simulink model "SOC_Estimation"  (R2024b)
settings: configuration reference "BMS_Sw_CodeGenConfig" (kept outside this file)
undefined symbols (not defined in the file): BatteryNN, BMS_State_Enum, DiscIntNeverNeededParam, Np_Module, Ns_Module, NumModules, SOCInit
libraries: simulink x1, BatteryEstimators x1
settings Model: DataDictionary=DD_SOC_Estimation.sldd  ExtModeTrigDuration=5  Creator=cpatel  LastModifiedBy=97433
settings ConfigSetRef: SourceName=BMS_Sw_CodeGenConfig

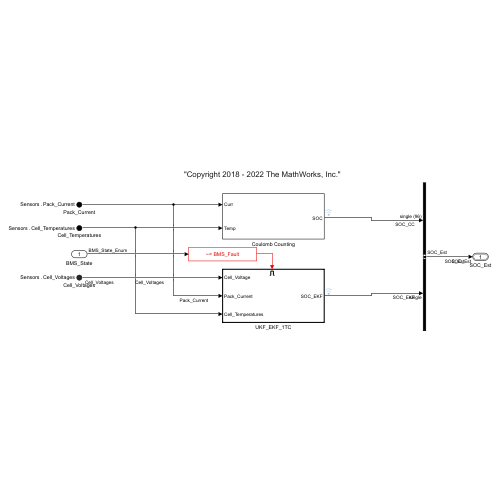
[thumbnail: Simulink's stored preview of the top-level diagram]
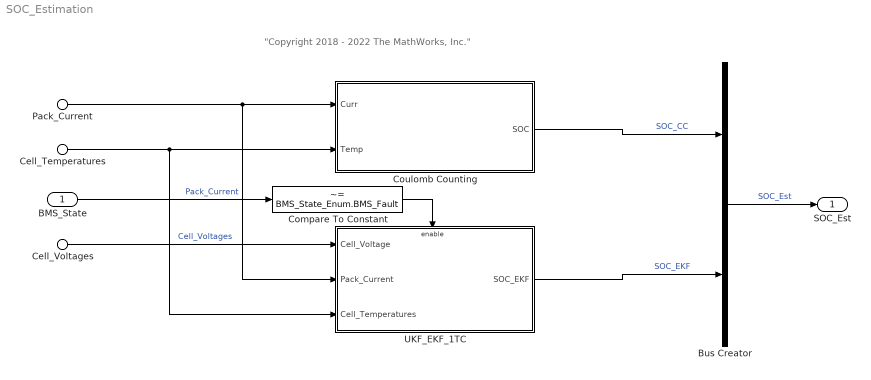
== system SOC_Estimation ==
  note: "Copyright 2018 - 2022 The MathWorks, Inc."
  BMS_State : Inport  OutDataTypeStr=Enum: BMS_State_Enum
  Cell_Voltages : Inport  Port=2  PortName=Sensors  Element=Cell_Voltages
  Pack_Current : Inport  Port=2  PortName=Sensors  Element=Pack_Current
  Cell_Temperatures : Inport  Port=2  PortName=Sensors  Element=Cell_Temperatures
  Bus Creator : BusCreator  Inputs=2  OutDataTypeStr=Bus: SOC_Est  NonVirtualBus=on
      settings: InheritFromInputs=off
  Compare To Constant : simulink/Logic and Bit Operations/Compare To Constant  relop=~=  const=BMS_State_Enum.BMS_Fault  OutDataTypeStr=boolean
  Coulomb Counting : Subsystem  VariantControl=SocAlgo==1
  UKF_EKF_1TC : Subsystem  VariantControl=CellType==1
  SOC_Est : Outport  OutDataTypeStr=Bus: SOC_Est  SampleTime=[0.10000000000000001,0]  VectorParamsAs1DForOutWhenUnconnected=off  BusOutputAsStruct=on
  wires:
  Cell_Voltages/1 -> UKF_EKF_1TC/1(Cell_Voltage)  "Cell_Voltages"
  Bus Creator/1 -> SOC_Est/1  "SOC_Est"
  Coulomb Counting/1(SOC) -> Bus Creator/1  "SOC_CC"
  UKF_EKF_1TC/1(SOC_EKF) -> Bus Creator/2  "SOC_EKF"
  BMS_State/1 -> Compare To Constant/1
  Compare To Constant/1 -> UKF_EKF_1TC/Enable
  Pack_Current/1 -> UKF_EKF_1TC/2(Pack_Current), Coulomb Counting/1(Curr)  "Pack_Current"
  Cell_Temperatures/1 -> Coulomb Counting/2(Temp), UKF_EKF_1TC/3(Cell_Temperatures)

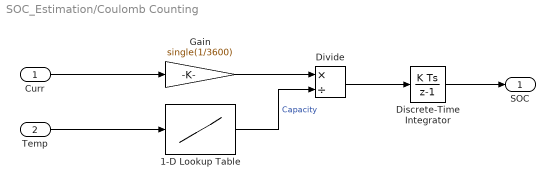
== system SOC_Estimation/Coulomb Counting ==
  Curr : Inport
  Temp : Inport  Port=2
  1-D Lookup Table : Lookup_n-D  NumberOfTableDimensions=1  BreakpointsForDimension1=single(BatteryNN(1).T_vec)  Table=single(BatteryNN(1).AH)*Np_Module  InternalRulePriority=Speed  RndMeth=Simplest
  Discrete-Time Integrator : DiscreteIntegrator  InitialCondition=ones(1,NumModules*Ns_Module)*single(SOCInit)  SampleTime=-1  LimitOutput=on  UpperSaturationLimit=1  LowerSaturationLimit=0  ICPrevOutput=DiscIntNeverNeededParam  ICPrevScaledInput=DiscIntNeverNeededParam
  Divide : Product  Inputs=*/
  Gain : Gain  Gain=single(1/3600)
  SOC : Outport  VectorParamsAs1DForOutWhenUnconnected=off
  wires:
  Discrete-Time Integrator/1 -> SOC/1
  Curr/1 -> Gain/1
  Gain/1 -> Divide/1
  Divide/1 -> Discrete-Time Integrator/1
  1-D Lookup Table/1 -> Divide/2  "Capacity"
  Temp/1 -> 1-D Lookup Table/1

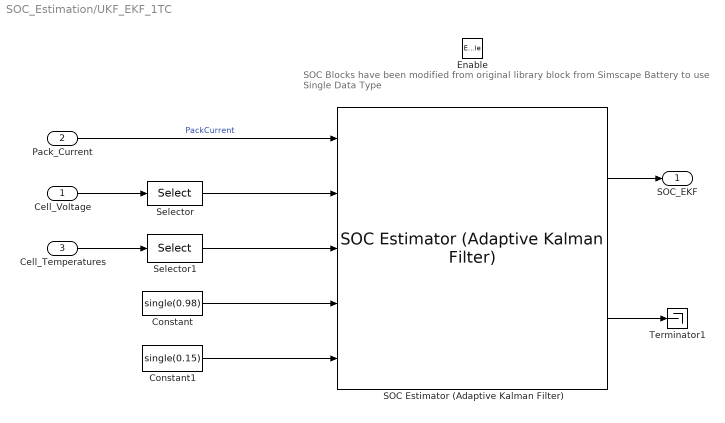
== system SOC_Estimation/UKF_EKF_1TC ==
  note: SOC Blocks have been modified from original library block from Simscape Battery
      | to use Single Data Type
  Cell_Voltage : Inport
  Pack_Current : Inport  Port=2
  Cell_Temperatures : Inport  Port=3
  Enable : EnablePort
  Constant : Constant  Value=single(0.98)
  Constant1 : Constant  Value=single(0.15)
  SOC Estimator (Adaptive Kalman Filter) : BatteryEstimators/SOC Estimator (Adaptive Kalman Filter)  CurrentInputPartition=off  filterType=Extended Kalman filter  alpha=1  beta=2  kappa=0  Q=|  Q_2RC=|  R=0.1  P0=[1e-5 0 0; 0 1 0; 0 0 1e-5]  P0_2RC="[1e-5 0 0 0; 0 1 0 0;0 0  1 0; 0 0 0 1e-5]"  Ts=-1  chargeDynamics=One time-constant dynamics  SOC_vec=[0, .1, .25, .5, .75, .9, 1]  T_vec=[278, 293, 313]  R1_mat=[.0109, .0029, .0013; .0069, .0024, .0012; .0047, .0026, .0013; .0034, .0016, .001; .0033, .0023, .0014; .0033, .0018, .0011; .0028, .0017, .0011]  tau1_mat=[20, 36, 39; 31, 45, 39; 109, 105, 61; 36, 29, 26; 59, 77, 67; 40, 33, 29; 25, 39, 33]  R2_mat=[.0109, .0029, .0013; .0069, .0024, .0012; .0047, .0026, .0013; .0034, .0016, .001; .0033, .0023, .0014; .0033, .0018, .0011; .0028, .0017, .0011]  tau2_mat=[20, 36, 39; 31, 45, 39; 109, 105, 61; 36, 29, 26; 59, 77, 67; 40, 33, 29; 25, 39, 33]  V0_mat=[3.49, 3.5, 3.51; 3.55, 3.57, 3.56; 3.62, 3.63, 3.64; 3.71, 3.71, 3.72; 3.91, 3.93, 3.94; 4.07, 4.08, 4.08; 4.19, 4.19, 4.19]  AH=27
      Q=|
      | [1e-6 0 0;
      | 0 1e-6 0;0 0 1e-6]
      Q_2RC=|
      | [1e-6 0 0 0;
      | 0 1e-6 0 0;0 0 1e-6 0;0 0 0 1e-6]
      settings: LibrarySourceBlock=|
      | batt_sl_lib/Estimators/SOC Estimator
      | (Adaptive Kalman Filter)
  Selector : Selector  InputPortWidth=Ns_Module*NumModules  IndexOptions=Starting index (dialog)  Indices=[1]  OutputSizes=1
  Selector1 : Selector  InputPortWidth=Ns_Module*NumModules  IndexOptions=Starting index (dialog)  Indices=[1]  OutputSizes=1
  Terminator1 : Terminator
  SOC_EKF : Outport  VectorParamsAs1DForOutWhenUnconnected=off
  wires:
  Pack_Current/1 -> SOC Estimator (Adaptive Kalman Filter)/1  "PackCurrent"
  SOC Estimator (Adaptive Kalman Filter)/2 -> Terminator1/1
  Cell_Temperatures/1 -> Selector1/1
  Cell_Voltage/1 -> Selector/1
  SOC Estimator (Adaptive Kalman Filter)/1 -> SOC_EKF/1
  Selector/1 -> SOC Estimator (Adaptive Kalman Filter)/2
  Selector1/1 -> SOC Estimator (Adaptive Kalman Filter)/3
  Constant/1 -> SOC Estimator (Adaptive Kalman Filter)/4
  Constant1/1 -> SOC Estimator (Adaptive Kalman Filter)/5
